simulink model "IOControls"  (R2019b)
settings: configuration reference "ConfigSet_IOControls_Reference" (kept outside this file)
model workspace (MAT data in the model file):
  SampleTime = 0.05
libraries: IOStateMachinesLib x274, SignalGeneratorsLib x1, simulink x1
(part 8 of 10)

== system IOControls/ForEachVehicle/IOControls/Non-CabControl/InteriorDoorControls/LeftDoor2ManualClose ==
  note: States:
      | Close
      | Open
  InputControl : Inport  OutDataTypeStr=Bus: BD_IOControls_In_InputControl
  Initialise : Inport  Port=2
  Bus Selector : BusSelector  OutputSignals=Value,Mode,InitVal,InternalRequest,Inhibit
  LeftDoor2ManualClose-Momentary : IOStateMachinesLib/Momentary  InitSource=internal  InitState=InitState
      settings: SourceProductName=IO State Machines
  InputState : Outport  VectorParamsAs1DForOutWhenUnconnected=off
  wires:
  Initialise/1 -> LeftDoor2ManualClose-Momentary/4
  LeftDoor2ManualClose-Momentary/1 -> InputState/1
  Bus Selector/5 -> LeftDoor2ManualClose-Momentary/6  "<Inhibit>"
  Bus Selector/4 -> LeftDoor2ManualClose-Momentary/5  "<InternalRequest>"
  Bus Selector/3 -> LeftDoor2ManualClose-Momentary/3  "<InitVal>"
  Bus Selector/2 -> LeftDoor2ManualClose-Momentary/2  "<Mode>"
  Bus Selector/1 -> LeftDoor2ManualClose-Momentary/1  "<Value>"
  InputControl/1 -> Bus Selector/1

== system IOControls/ForEachVehicle/IOControls/Non-CabControl/InteriorDoorControls/LeftDoor2ManualOpen ==
  note: States:
      | Close
      | Open
  InputControl : Inport  OutDataTypeStr=Bus: BD_IOControls_In_InputControl
  Initialise : Inport  Port=2
  Bus Selector : BusSelector  OutputSignals=Value,Mode,InitVal,InternalRequest,Inhibit
  LeftDoor2ManualOpen-Momentary : IOStateMachinesLib/Momentary  InitSource=internal  InitState=InitState
      settings: SourceProductName=IO State Machines
  InputState : Outport  VectorParamsAs1DForOutWhenUnconnected=off
  wires:
  Initialise/1 -> LeftDoor2ManualOpen-Momentary/4
  LeftDoor2ManualOpen-Momentary/1 -> InputState/1
  Bus Selector/5 -> LeftDoor2ManualOpen-Momentary/6  "<Inhibit>"
  Bus Selector/4 -> LeftDoor2ManualOpen-Momentary/5  "<InternalRequest>"
  Bus Selector/3 -> LeftDoor2ManualOpen-Momentary/3  "<InitVal>"
  Bus Selector/2 -> LeftDoor2ManualOpen-Momentary/2  "<Mode>"
  Bus Selector/1 -> LeftDoor2ManualOpen-Momentary/1  "<Value>"
  InputControl/1 -> Bus Selector/1

== system IOControls/ForEachVehicle/IOControls/Non-CabControl/InteriorDoorControls/LeftDoor3Coving ==
  note: States:
      | Closed
      | Open
  InputControl : Inport  OutDataTypeStr=Bus: BD_IOControls_In_InputControl
  Initialise : Inport  Port=2
  Bus Selector : BusSelector  OutputSignals=Value,Mode,InitVal,InternalRequest,Inhibit
  LeftDoor3Coving-Toggle : IOStateMachinesLib/Toggle  InitSource=internal  InitState=InitState  OffStateValue=OffStateValue  OnStateValue=OnStateValue
      settings: SourceProductName=IO State Machines
  InputState : Outport  VectorParamsAs1DForOutWhenUnconnected=off
  wires:
  Initialise/1 -> LeftDoor3Coving-Toggle/4
  LeftDoor3Coving-Toggle/1 -> InputState/1
  Bus Selector/5 -> LeftDoor3Coving-Toggle/6  "<Inhibit>"
  Bus Selector/4 -> LeftDoor3Coving-Toggle/5  "<InternalRequest>"
  Bus Selector/3 -> LeftDoor3Coving-Toggle/3  "<InitVal>"
  Bus Selector/2 -> LeftDoor3Coving-Toggle/2  "<Mode>"
  Bus Selector/1 -> LeftDoor3Coving-Toggle/1  "<Value>"
  InputControl/1 -> Bus Selector/1

== system IOControls/ForEachVehicle/IOControls/Non-CabControl/InteriorDoorControls/LeftDoor3DCUCB ==
  note: States:
      | Tripped
      | Set
  MCBControl : Inport  OutDataTypeStr=Bus: BD_IOControls_In_MCBControl
  Initialise : Inport  Port=2
  Bus Selector : BusSelector  OutputSignals=Value,Mode,InitVal,InternalRequest,Inhibit,TripRequest
  LeftDoor3DCUCB-MCB : IOStateMachinesLib/MCB  InitSource=internal  InitState=InitState  OffStateValue=OffStateValue  OnStateValue=OnStateValue
      settings: SourceProductName=IO State Machines
  InputState : Outport  VectorParamsAs1DForOutWhenUnconnected=off
  MCBTripState : Outport  Port=2  VectorParamsAs1DForOutWhenUnconnected=off
  wires:
  LeftDoor3DCUCB-MCB/2 -> MCBTripState/1
  Bus Selector/6 -> LeftDoor3DCUCB-MCB/7  "<TripRequest>"
  MCBControl/1 -> Bus Selector/1
  Bus Selector/1 -> LeftDoor3DCUCB-MCB/1  "<Value>"
  Bus Selector/2 -> LeftDoor3DCUCB-MCB/2  "<Mode>"
  Bus Selector/3 -> LeftDoor3DCUCB-MCB/3  "<InitVal>"
  Bus Selector/4 -> LeftDoor3DCUCB-MCB/5  "<InternalRequest>"
  Bus Selector/5 -> LeftDoor3DCUCB-MCB/6  "<Inhibit>"
  LeftDoor3DCUCB-MCB/1 -> InputState/1
  Initialise/1 -> LeftDoor3DCUCB-MCB/4

== system IOControls/ForEachVehicle/IOControls/Non-CabControl/InteriorDoorControls/LeftDoor3EED ==
  note: States:
      | Reset
      | Operated
  InputControl : Inport  OutDataTypeStr=Bus: BD_IOControls_In_InputControl
  Initialise : Inport  Port=2
  Bus Selector : BusSelector  OutputSignals=Value,Mode,InitVal,InternalRequest,Inhibit
  LeftDoor3EED-Momentary : IOStateMachinesLib/Momentary  InitSource=internal  InitState=InitState
      settings: SourceProductName=IO State Machines
  InputState : Outport  VectorParamsAs1DForOutWhenUnconnected=off
  wires:
  Initialise/1 -> LeftDoor3EED-Momentary/4
  LeftDoor3EED-Momentary/1 -> InputState/1
  Bus Selector/5 -> LeftDoor3EED-Momentary/6  "<Inhibit>"
  Bus Selector/4 -> LeftDoor3EED-Momentary/5  "<InternalRequest>"
  Bus Selector/3 -> LeftDoor3EED-Momentary/3  "<InitVal>"
  Bus Selector/2 -> LeftDoor3EED-Momentary/2  "<Mode>"
  Bus Selector/1 -> LeftDoor3EED-Momentary/1  "<Value>"
  InputControl/1 -> Bus Selector/1

== system IOControls/ForEachVehicle/IOControls/Non-CabControl/InteriorDoorControls/LeftDoor3Lockout ==
  note: States:
      | Unlocked
      | Locked
  InputControl : Inport  OutDataTypeStr=Bus: BD_IOControls_In_InputControl
  Initialise : Inport  Port=2
  Bus Selector : BusSelector  OutputSignals=Value,Mode,InitVal,InternalRequest,Inhibit
  LeftDoor3Lockout-Toggle : IOStateMachinesLib/Toggle  InitSource=internal  InitState=InitState  OffStateValue=OffStateValue  OnStateValue=OnStateValue
      settings: SourceProductName=IO State Machines
  InputState : Outport  VectorParamsAs1DForOutWhenUnconnected=off
  wires:
  Initialise/1 -> LeftDoor3Lockout-Toggle/4
  LeftDoor3Lockout-Toggle/1 -> InputState/1
  Bus Selector/5 -> LeftDoor3Lockout-Toggle/6  "<Inhibit>"
  Bus Selector/4 -> LeftDoor3Lockout-Toggle/5  "<InternalRequest>"
  Bus Selector/3 -> LeftDoor3Lockout-Toggle/3  "<InitVal>"
  Bus Selector/2 -> LeftDoor3Lockout-Toggle/2  "<Mode>"
  Bus Selector/1 -> LeftDoor3Lockout-Toggle/1  "<Value>"
  InputControl/1 -> Bus Selector/1

== system IOControls/ForEachVehicle/IOControls/Non-CabControl/InteriorDoorControls/LeftDoor3ManualClose ==
  note: States:
      | Close
      | Open
  InputControl : Inport  OutDataTypeStr=Bus: BD_IOControls_In_InputControl
  Initialise : Inport  Port=2
  Bus Selector : BusSelector  OutputSignals=Value,Mode,InitVal,InternalRequest,Inhibit
  LeftDoor3ManualClose-Momentary : IOStateMachinesLib/Momentary  InitSource=internal  InitState=InitState
      settings: SourceProductName=IO State Machines
  InputState : Outport  VectorParamsAs1DForOutWhenUnconnected=off
  wires:
  Initialise/1 -> LeftDoor3ManualClose-Momentary/4
  LeftDoor3ManualClose-Momentary/1 -> InputState/1
  Bus Selector/5 -> LeftDoor3ManualClose-Momentary/6  "<Inhibit>"
  Bus Selector/4 -> LeftDoor3ManualClose-Momentary/5  "<InternalRequest>"
  Bus Selector/3 -> LeftDoor3ManualClose-Momentary/3  "<InitVal>"
  Bus Selector/2 -> LeftDoor3ManualClose-Momentary/2  "<Mode>"
  Bus Selector/1 -> LeftDoor3ManualClose-Momentary/1  "<Value>"
  InputControl/1 -> Bus Selector/1

== system IOControls/ForEachVehicle/IOControls/Non-CabControl/InteriorDoorControls/LeftDoor3ManualOpen ==
  note: States:
      | Close
      | Open
  InputControl : Inport  OutDataTypeStr=Bus: BD_IOControls_In_InputControl
  Initialise : Inport  Port=2
  Bus Selector : BusSelector  OutputSignals=Value,Mode,InitVal,InternalRequest,Inhibit
  LeftDoor3ManualOpen-Momentary : IOStateMachinesLib/Momentary  InitSource=internal  InitState=InitState
      settings: SourceProductName=IO State Machines
  InputState : Outport  VectorParamsAs1DForOutWhenUnconnected=off
  wires:
  Initialise/1 -> LeftDoor3ManualOpen-Momentary/4
  LeftDoor3ManualOpen-Momentary/1 -> InputState/1
  Bus Selector/5 -> LeftDoor3ManualOpen-Momentary/6  "<Inhibit>"
  Bus Selector/4 -> LeftDoor3ManualOpen-Momentary/5  "<InternalRequest>"
  Bus Selector/3 -> LeftDoor3ManualOpen-Momentary/3  "<InitVal>"
  Bus Selector/2 -> LeftDoor3ManualOpen-Momentary/2  "<Mode>"
  Bus Selector/1 -> LeftDoor3ManualOpen-Momentary/1  "<Value>"
  InputControl/1 -> Bus Selector/1

== system IOControls/ForEachVehicle/IOControls/Non-CabControl/InteriorDoorControls/LeftDoor4Coving ==
  note: States:
      | Closed
      | Open
  InputControl : Inport  OutDataTypeStr=Bus: BD_IOControls_In_InputControl
  Initialise : Inport  Port=2
  Bus Selector : BusSelector  OutputSignals=Value,Mode,InitVal,InternalRequest,Inhibit
  LeftDoor4Coving-Toggle : IOStateMachinesLib/Toggle  InitSource=internal  InitState=InitState  OffStateValue=OffStateValue  OnStateValue=OnStateValue
      settings: SourceProductName=IO State Machines
  InputState : Outport  VectorParamsAs1DForOutWhenUnconnected=off
  wires:
  Initialise/1 -> LeftDoor4Coving-Toggle/4
  LeftDoor4Coving-Toggle/1 -> InputState/1
  Bus Selector/5 -> LeftDoor4Coving-Toggle/6  "<Inhibit>"
  Bus Selector/4 -> LeftDoor4Coving-Toggle/5  "<InternalRequest>"
  Bus Selector/3 -> LeftDoor4Coving-Toggle/3  "<InitVal>"
  Bus Selector/2 -> LeftDoor4Coving-Toggle/2  "<Mode>"
  Bus Selector/1 -> LeftDoor4Coving-Toggle/1  "<Value>"
  InputControl/1 -> Bus Selector/1

== system IOControls/ForEachVehicle/IOControls/Non-CabControl/InteriorDoorControls/LeftDoor4DCUCB ==
  note: States:
      | Tripped
      | Set
  MCBControl : Inport  OutDataTypeStr=Bus: BD_IOControls_In_MCBControl
  Initialise : Inport  Port=2
  Bus Selector : BusSelector  OutputSignals=Value,Mode,InitVal,InternalRequest,Inhibit,TripRequest
  LeftDoor4DCUCB-MCB : IOStateMachinesLib/MCB  InitSource=internal  InitState=InitState  OffStateValue=OffStateValue  OnStateValue=OnStateValue
      settings: SourceProductName=IO State Machines
  InputState : Outport  VectorParamsAs1DForOutWhenUnconnected=off
  MCBTripState : Outport  Port=2  VectorParamsAs1DForOutWhenUnconnected=off
  wires:
  LeftDoor4DCUCB-MCB/2 -> MCBTripState/1
  Bus Selector/6 -> LeftDoor4DCUCB-MCB/7  "<TripRequest>"
  MCBControl/1 -> Bus Selector/1
  Bus Selector/1 -> LeftDoor4DCUCB-MCB/1  "<Value>"
  Bus Selector/2 -> LeftDoor4DCUCB-MCB/2  "<Mode>"
  Bus Selector/3 -> LeftDoor4DCUCB-MCB/3  "<InitVal>"
  Bus Selector/4 -> LeftDoor4DCUCB-MCB/5  "<InternalRequest>"
  Bus Selector/5 -> LeftDoor4DCUCB-MCB/6  "<Inhibit>"
  LeftDoor4DCUCB-MCB/1 -> InputState/1
  Initialise/1 -> LeftDoor4DCUCB-MCB/4

== system IOControls/ForEachVehicle/IOControls/Non-CabControl/InteriorDoorControls/LeftDoor4EED ==
  note: States:
      | Reset
      | Operated
  InputControl : Inport  OutDataTypeStr=Bus: BD_IOControls_In_InputControl
  Initialise : Inport  Port=2
  Bus Selector : BusSelector  OutputSignals=Value,Mode,InitVal,InternalRequest,Inhibit
  LeftDoor4EED-Momentary : IOStateMachinesLib/Momentary  InitSource=internal  InitState=InitState
      settings: SourceProductName=IO State Machines
  InputState : Outport  VectorParamsAs1DForOutWhenUnconnected=off
  wires:
  Initialise/1 -> LeftDoor4EED-Momentary/4
  LeftDoor4EED-Momentary/1 -> InputState/1
  Bus Selector/5 -> LeftDoor4EED-Momentary/6  "<Inhibit>"
  Bus Selector/4 -> LeftDoor4EED-Momentary/5  "<InternalRequest>"
  Bus Selector/3 -> LeftDoor4EED-Momentary/3  "<InitVal>"
  Bus Selector/2 -> LeftDoor4EED-Momentary/2  "<Mode>"
  Bus Selector/1 -> LeftDoor4EED-Momentary/1  "<Value>"
  InputControl/1 -> Bus Selector/1

== system IOControls/ForEachVehicle/IOControls/Non-CabControl/InteriorDoorControls/LeftDoor4Lockout ==
  note: States:
      | Unlocked
      | Locked
  InputControl : Inport  OutDataTypeStr=Bus: BD_IOControls_In_InputControl
  Initialise : Inport  Port=2
  Bus Selector : BusSelector  OutputSignals=Value,Mode,InitVal,InternalRequest,Inhibit
  LeftDoor4Lockout-Toggle : IOStateMachinesLib/Toggle  InitSource=internal  InitState=InitState  OffStateValue=OffStateValue  OnStateValue=OnStateValue
      settings: SourceProductName=IO State Machines
  InputState : Outport  VectorParamsAs1DForOutWhenUnconnected=off
  wires:
  Initialise/1 -> LeftDoor4Lockout-Toggle/4
  LeftDoor4Lockout-Toggle/1 -> InputState/1
  Bus Selector/5 -> LeftDoor4Lockout-Toggle/6  "<Inhibit>"
  Bus Selector/4 -> LeftDoor4Lockout-Toggle/5  "<InternalRequest>"
  Bus Selector/3 -> LeftDoor4Lockout-Toggle/3  "<InitVal>"
  Bus Selector/2 -> LeftDoor4Lockout-Toggle/2  "<Mode>"
  Bus Selector/1 -> LeftDoor4Lockout-Toggle/1  "<Value>"
  InputControl/1 -> Bus Selector/1

== system IOControls/ForEachVehicle/IOControls/Non-CabControl/InteriorDoorControls/LeftDoor4ManualClose ==
  note: States:
      | Close
      | Open
  InputControl : Inport  OutDataTypeStr=Bus: BD_IOControls_In_InputControl
  Initialise : Inport  Port=2
  Bus Selector : BusSelector  OutputSignals=Value,Mode,InitVal,InternalRequest,Inhibit
  LeftDoor4ManualClose-Momentary : IOStateMachinesLib/Momentary  InitSource=internal  InitState=InitState
      settings: SourceProductName=IO State Machines
  InputState : Outport  VectorParamsAs1DForOutWhenUnconnected=off
  wires:
  Initialise/1 -> LeftDoor4ManualClose-Momentary/4
  LeftDoor4ManualClose-Momentary/1 -> InputState/1
  Bus Selector/5 -> LeftDoor4ManualClose-Momentary/6  "<Inhibit>"
  Bus Selector/4 -> LeftDoor4ManualClose-Momentary/5  "<InternalRequest>"
  Bus Selector/3 -> LeftDoor4ManualClose-Momentary/3  "<InitVal>"
  Bus Selector/2 -> LeftDoor4ManualClose-Momentary/2  "<Mode>"
  Bus Selector/1 -> LeftDoor4ManualClose-Momentary/1  "<Value>"
  InputControl/1 -> Bus Selector/1

== system IOControls/ForEachVehicle/IOControls/Non-CabControl/InteriorDoorControls/LeftDoor4ManualOpen ==
  note: States:
      | Close
      | Open
  InputControl : Inport  OutDataTypeStr=Bus: BD_IOControls_In_InputControl
  Initialise : Inport  Port=2
  Bus Selector : BusSelector  OutputSignals=Value,Mode,InitVal,InternalRequest,Inhibit
  LeftDoor4ManualOpen-Momentary : IOStateMachinesLib/Momentary  InitSource=internal  InitState=InitState
      settings: SourceProductName=IO State Machines
  InputState : Outport  VectorParamsAs1DForOutWhenUnconnected=off
  wires:
  Initialise/1 -> LeftDoor4ManualOpen-Momentary/4
  LeftDoor4ManualOpen-Momentary/1 -> InputState/1
  Bus Selector/5 -> LeftDoor4ManualOpen-Momentary/6  "<Inhibit>"
  Bus Selector/4 -> LeftDoor4ManualOpen-Momentary/5  "<InternalRequest>"
  Bus Selector/3 -> LeftDoor4ManualOpen-Momentary/3  "<InitVal>"
  Bus Selector/2 -> LeftDoor4ManualOpen-Momentary/2  "<Mode>"
  Bus Selector/1 -> LeftDoor4ManualOpen-Momentary/1  "<Value>"
  InputControl/1 -> Bus Selector/1

== system IOControls/ForEachVehicle/IOControls/Non-CabControl/InteriorDoorControls/RightDoor1Coving ==
  note: States:
      | Closed
      | Open
  InputControl : Inport  OutDataTypeStr=Bus: BD_IOControls_In_InputControl
  Initialise : Inport  Port=2
  Bus Selector : BusSelector  OutputSignals=Value,Mode,InitVal,InternalRequest,Inhibit
  RightDoor1Coving-Toggle : IOStateMachinesLib/Toggle  InitSource=internal  InitState=InitState  OffStateValue=OffStateValue  OnStateValue=OnStateValue
      settings: SourceProductName=IO State Machines
  InputState : Outport  VectorParamsAs1DForOutWhenUnconnected=off
  wires:
  Initialise/1 -> RightDoor1Coving-Toggle/4
  RightDoor1Coving-Toggle/1 -> InputState/1
  Bus Selector/5 -> RightDoor1Coving-Toggle/6  "<Inhibit>"
  Bus Selector/4 -> RightDoor1Coving-Toggle/5  "<InternalRequest>"
  Bus Selector/3 -> RightDoor1Coving-Toggle/3  "<InitVal>"
  Bus Selector/2 -> RightDoor1Coving-Toggle/2  "<Mode>"
  Bus Selector/1 -> RightDoor1Coving-Toggle/1  "<Value>"
  InputControl/1 -> Bus Selector/1

== system IOControls/ForEachVehicle/IOControls/Non-CabControl/InteriorDoorControls/RightDoor1DCUCB ==
  note: States:
      | Tripped
      | Set
  MCBControl : Inport  OutDataTypeStr=Bus: BD_IOControls_In_MCBControl
  Initialise : Inport  Port=2
  Bus Selector : BusSelector  OutputSignals=Value,Mode,InitVal,InternalRequest,Inhibit,TripRequest
  RightDoor1DCUCB-MCB : IOStateMachinesLib/MCB  InitSource=internal  InitState=InitState  OffStateValue=OffStateValue  OnStateValue=OnStateValue
      settings: SourceProductName=IO State Machines
  InputState : Outport  VectorParamsAs1DForOutWhenUnconnected=off
  MCBTripState : Outport  Port=2  VectorParamsAs1DForOutWhenUnconnected=off
  wires:
  RightDoor1DCUCB-MCB/2 -> MCBTripState/1
  Bus Selector/6 -> RightDoor1DCUCB-MCB/7  "<TripRequest>"
  MCBControl/1 -> Bus Selector/1
  Bus Selector/1 -> RightDoor1DCUCB-MCB/1  "<Value>"
  Bus Selector/2 -> RightDoor1DCUCB-MCB/2  "<Mode>"
  Bus Selector/3 -> RightDoor1DCUCB-MCB/3  "<InitVal>"
  Bus Selector/4 -> RightDoor1DCUCB-MCB/5  "<InternalRequest>"
  Bus Selector/5 -> RightDoor1DCUCB-MCB/6  "<Inhibit>"
  RightDoor1DCUCB-MCB/1 -> InputState/1
  Initialise/1 -> RightDoor1DCUCB-MCB/4

== system IOControls/ForEachVehicle/IOControls/Non-CabControl/InteriorDoorControls/RightDoor1EED ==
  note: States:
      | Reset
      | Operated
  InputControl : Inport  OutDataTypeStr=Bus: BD_IOControls_In_InputControl
  Initialise : Inport  Port=2
  Bus Selector : BusSelector  OutputSignals=Value,Mode,InitVal,InternalRequest,Inhibit
  RightDoor1EED-Momentary : IOStateMachinesLib/Momentary  InitSource=internal  InitState=InitState
      settings: SourceProductName=IO State Machines
  InputState : Outport  VectorParamsAs1DForOutWhenUnconnected=off
  wires:
  Initialise/1 -> RightDoor1EED-Momentary/4
  RightDoor1EED-Momentary/1 -> InputState/1
  Bus Selector/5 -> RightDoor1EED-Momentary/6  "<Inhibit>"
  Bus Selector/4 -> RightDoor1EED-Momentary/5  "<InternalRequest>"
  Bus Selector/3 -> RightDoor1EED-Momentary/3  "<InitVal>"
  Bus Selector/2 -> RightDoor1EED-Momentary/2  "<Mode>"
  Bus Selector/1 -> RightDoor1EED-Momentary/1  "<Value>"
  InputControl/1 -> Bus Selector/1

== system IOControls/ForEachVehicle/IOControls/Non-CabControl/InteriorDoorControls/RightDoor1Lockout ==
  note: States:
      | Unlocked
      | Locked
  InputControl : Inport  OutDataTypeStr=Bus: BD_IOControls_In_InputControl
  Initialise : Inport  Port=2
  Bus Selector : BusSelector  OutputSignals=Value,Mode,InitVal,InternalRequest,Inhibit
  RightDoor1Lockout-Toggle : IOStateMachinesLib/Toggle  InitSource=internal  InitState=InitState  OffStateValue=OffStateValue  OnStateValue=OnStateValue
      settings: SourceProductName=IO State Machines
  InputState : Outport  VectorParamsAs1DForOutWhenUnconnected=off
  wires:
  Initialise/1 -> RightDoor1Lockout-Toggle/4
  RightDoor1Lockout-Toggle/1 -> InputState/1
  Bus Selector/5 -> RightDoor1Lockout-Toggle/6  "<Inhibit>"
  Bus Selector/4 -> RightDoor1Lockout-Toggle/5  "<InternalRequest>"
  Bus Selector/3 -> RightDoor1Lockout-Toggle/3  "<InitVal>"
  Bus Selector/2 -> RightDoor1Lockout-Toggle/2  "<Mode>"
  Bus Selector/1 -> RightDoor1Lockout-Toggle/1  "<Value>"
  InputControl/1 -> Bus Selector/1

== system IOControls/ForEachVehicle/IOControls/Non-CabControl/InteriorDoorControls/RightDoor1ManualClose ==
  note: States:
      | Close
      | Open
  InputControl : Inport  OutDataTypeStr=Bus: BD_IOControls_In_InputControl
  Initialise : Inport  Port=2
  Bus Selector : BusSelector  OutputSignals=Value,Mode,InitVal,InternalRequest,Inhibit
  RightDoor1ManualClose-Momentary : IOStateMachinesLib/Momentary  InitSource=internal  InitState=InitState
      settings: SourceProductName=IO State Machines
  InputState : Outport  VectorParamsAs1DForOutWhenUnconnected=off
  wires:
  Initialise/1 -> RightDoor1ManualClose-Momentary/4
  RightDoor1ManualClose-Momentary/1 -> InputState/1
  Bus Selector/5 -> RightDoor1ManualClose-Momentary/6  "<Inhibit>"
  Bus Selector/4 -> RightDoor1ManualClose-Momentary/5  "<InternalRequest>"
  Bus Selector/3 -> RightDoor1ManualClose-Momentary/3  "<InitVal>"
  Bus Selector/2 -> RightDoor1ManualClose-Momentary/2  "<Mode>"
  Bus Selector/1 -> RightDoor1ManualClose-Momentary/1  "<Value>"
  InputControl/1 -> Bus Selector/1

== system IOControls/ForEachVehicle/IOControls/Non-CabControl/InteriorDoorControls/RightDoor1ManualOpen ==
  note: States:
      | Close
      | Open
  InputControl : Inport  OutDataTypeStr=Bus: BD_IOControls_In_InputControl
  Initialise : Inport  Port=2
  Bus Selector : BusSelector  OutputSignals=Value,Mode,InitVal,InternalRequest,Inhibit
  RightDoor1ManualOpen-Momentary : IOStateMachinesLib/Momentary  InitSource=internal  InitState=InitState
      settings: SourceProductName=IO State Machines
  InputState : Outport  VectorParamsAs1DForOutWhenUnconnected=off
  wires:
  Initialise/1 -> RightDoor1ManualOpen-Momentary/4
  RightDoor1ManualOpen-Momentary/1 -> InputState/1
  Bus Selector/5 -> RightDoor1ManualOpen-Momentary/6  "<Inhibit>"
  Bus Selector/4 -> RightDoor1ManualOpen-Momentary/5  "<InternalRequest>"
  Bus Selector/3 -> RightDoor1ManualOpen-Momentary/3  "<InitVal>"
  Bus Selector/2 -> RightDoor1ManualOpen-Momentary/2  "<Mode>"
  Bus Selector/1 -> RightDoor1ManualOpen-Momentary/1  "<Value>"
  InputControl/1 -> Bus Selector/1

== system IOControls/ForEachVehicle/IOControls/Non-CabControl/InteriorDoorControls/RightDoor2Coving ==
  note: States:
      | Closed
      | Open
  InputControl : Inport  OutDataTypeStr=Bus: BD_IOControls_In_InputControl
  Initialise : Inport  Port=2
  Bus Selector : BusSelector  OutputSignals=Value,Mode,InitVal,InternalRequest,Inhibit
  RightDoor2Coving-Toggle : IOStateMachinesLib/Toggle  InitSource=internal  InitState=InitState  OffStateValue=OffStateValue  OnStateValue=OnStateValue
      settings: SourceProductName=IO State Machines
  InputState : Outport  VectorParamsAs1DForOutWhenUnconnected=off
  wires:
  Initialise/1 -> RightDoor2Coving-Toggle/4
  RightDoor2Coving-Toggle/1 -> InputState/1
  Bus Selector/5 -> RightDoor2Coving-Toggle/6  "<Inhibit>"
  Bus Selector/4 -> RightDoor2Coving-Toggle/5  "<InternalRequest>"
  Bus Selector/3 -> RightDoor2Coving-Toggle/3  "<InitVal>"
  Bus Selector/2 -> RightDoor2Coving-Toggle/2  "<Mode>"
  Bus Selector/1 -> RightDoor2Coving-Toggle/1  "<Value>"
  InputControl/1 -> Bus Selector/1

== system IOControls/ForEachVehicle/IOControls/Non-CabControl/InteriorDoorControls/RightDoor2DCUCB ==
  note: States:
      | Tripped
      | Set
  MCBControl : Inport  OutDataTypeStr=Bus: BD_IOControls_In_MCBControl
  Initialise : Inport  Port=2
  Bus Selector : BusSelector  OutputSignals=Value,Mode,InitVal,InternalRequest,Inhibit,TripRequest
  RightDoor2DCUCB-MCB : IOStateMachinesLib/MCB  InitSource=internal  InitState=InitState  OffStateValue=OffStateValue  OnStateValue=OnStateValue
      settings: SourceProductName=IO State Machines
  InputState : Outport  VectorParamsAs1DForOutWhenUnconnected=off
  MCBTripState : Outport  Port=2  VectorParamsAs1DForOutWhenUnconnected=off
  wires:
  RightDoor2DCUCB-MCB/2 -> MCBTripState/1
  Bus Selector/6 -> RightDoor2DCUCB-MCB/7  "<TripRequest>"
  MCBControl/1 -> Bus Selector/1
  Bus Selector/1 -> RightDoor2DCUCB-MCB/1  "<Value>"
  Bus Selector/2 -> RightDoor2DCUCB-MCB/2  "<Mode>"
  Bus Selector/3 -> RightDoor2DCUCB-MCB/3  "<InitVal>"
  Bus Selector/4 -> RightDoor2DCUCB-MCB/5  "<InternalRequest>"
  Bus Selector/5 -> RightDoor2DCUCB-MCB/6  "<Inhibit>"
  RightDoor2DCUCB-MCB/1 -> InputState/1
  Initialise/1 -> RightDoor2DCUCB-MCB/4

== system IOControls/ForEachVehicle/IOControls/Non-CabControl/InteriorDoorControls/RightDoor2EED ==
  note: States:
      | Reset
      | Operated
  InputControl : Inport  OutDataTypeStr=Bus: BD_IOControls_In_InputControl
  Initialise : Inport  Port=2
  Bus Selector : BusSelector  OutputSignals=Value,Mode,InitVal,InternalRequest,Inhibit
  RightDoor2EED-Momentary : IOStateMachinesLib/Momentary  InitSource=internal  InitState=InitState
      settings: SourceProductName=IO State Machines
  InputState : Outport  VectorParamsAs1DForOutWhenUnconnected=off
  wires:
  Initialise/1 -> RightDoor2EED-Momentary/4
  RightDoor2EED-Momentary/1 -> InputState/1
  Bus Selector/5 -> RightDoor2EED-Momentary/6  "<Inhibit>"
  Bus Selector/4 -> RightDoor2EED-Momentary/5  "<InternalRequest>"
  Bus Selector/3 -> RightDoor2EED-Momentary/3  "<InitVal>"
  Bus Selector/2 -> RightDoor2EED-Momentary/2  "<Mode>"
  Bus Selector/1 -> RightDoor2EED-Momentary/1  "<Value>"
  InputControl/1 -> Bus Selector/1

== system IOControls/ForEachVehicle/IOControls/Non-CabControl/InteriorDoorControls/RightDoor2Lockout ==
  note: States:
      | Unlocked
      | Locked
  InputControl : Inport  OutDataTypeStr=Bus: BD_IOControls_In_InputControl
  Initialise : Inport  Port=2
  Bus Selector : BusSelector  OutputSignals=Value,Mode,InitVal,InternalRequest,Inhibit
  RightDoor2Lockout-Toggle : IOStateMachinesLib/Toggle  InitSource=internal  InitState=InitState  OffStateValue=OffStateValue  OnStateValue=OnStateValue
      settings: SourceProductName=IO State Machines
  InputState : Outport  VectorParamsAs1DForOutWhenUnconnected=off
  wires:
  Initialise/1 -> RightDoor2Lockout-Toggle/4
  RightDoor2Lockout-Toggle/1 -> InputState/1
  Bus Selector/5 -> RightDoor2Lockout-Toggle/6  "<Inhibit>"
  Bus Selector/4 -> RightDoor2Lockout-Toggle/5  "<InternalRequest>"
  Bus Selector/3 -> RightDoor2Lockout-Toggle/3  "<InitVal>"
  Bus Selector/2 -> RightDoor2Lockout-Toggle/2  "<Mode>"
  Bus Selector/1 -> RightDoor2Lockout-Toggle/1  "<Value>"
  InputControl/1 -> Bus Selector/1

== system IOControls/ForEachVehicle/IOControls/Non-CabControl/InteriorDoorControls/RightDoor2ManualClose ==
  note: States:
      | Close
      | Open
  InputControl : Inport  OutDataTypeStr=Bus: BD_IOControls_In_InputControl
  Initialise : Inport  Port=2
  Bus Selector : BusSelector  OutputSignals=Value,Mode,InitVal,InternalRequest,Inhibit
  RightDoor2ManualClose-Momentary : IOStateMachinesLib/Momentary  InitSource=internal  InitState=InitState
      settings: SourceProductName=IO State Machines
  InputState : Outport  VectorParamsAs1DForOutWhenUnconnected=off
  wires:
  Initialise/1 -> RightDoor2ManualClose-Momentary/4
  RightDoor2ManualClose-Momentary/1 -> InputState/1
  Bus Selector/5 -> RightDoor2ManualClose-Momentary/6  "<Inhibit>"
  Bus Selector/4 -> RightDoor2ManualClose-Momentary/5  "<InternalRequest>"
  Bus Selector/3 -> RightDoor2ManualClose-Momentary/3  "<InitVal>"
  Bus Selector/2 -> RightDoor2ManualClose-Momentary/2  "<Mode>"
  Bus Selector/1 -> RightDoor2ManualClose-Momentary/1  "<Value>"
  InputControl/1 -> Bus Selector/1

== system IOControls/ForEachVehicle/IOControls/Non-CabControl/InteriorDoorControls/RightDoor2ManualOpen ==
  note: States:
      | Close
      | Open
  InputControl : Inport  OutDataTypeStr=Bus: BD_IOControls_In_InputControl
  Initialise : Inport  Port=2
  Bus Selector : BusSelector  OutputSignals=Value,Mode,InitVal,InternalRequest,Inhibit
  RightDoor2ManualOpen-Momentary : IOStateMachinesLib/Momentary  InitSource=internal  InitState=InitState
      settings: SourceProductName=IO State Machines
  InputState : Outport  VectorParamsAs1DForOutWhenUnconnected=off
  wires:
  Initialise/1 -> RightDoor2ManualOpen-Momentary/4
  RightDoor2ManualOpen-Momentary/1 -> InputState/1
  Bus Selector/5 -> RightDoor2ManualOpen-Momentary/6  "<Inhibit>"
  Bus Selector/4 -> RightDoor2ManualOpen-Momentary/5  "<InternalRequest>"
  Bus Selector/3 -> RightDoor2ManualOpen-Momentary/3  "<InitVal>"
  Bus Selector/2 -> RightDoor2ManualOpen-Momentary/2  "<Mode>"
  Bus Selector/1 -> RightDoor2ManualOpen-Momentary/1  "<Value>"
  InputControl/1 -> Bus Selector/1

== system IOControls/ForEachVehicle/IOControls/Non-CabControl/InteriorDoorControls/RightDoor3Coving ==
  note: States:
      | Closed
      | Open
  InputControl : Inport  OutDataTypeStr=Bus: BD_IOControls_In_InputControl
  Initialise : Inport  Port=2
  Bus Selector : BusSelector  OutputSignals=Value,Mode,InitVal,InternalRequest,Inhibit
  RightDoor3Coving-Toggle : IOStateMachinesLib/Toggle  InitSource=internal  InitState=InitState  OffStateValue=OffStateValue  OnStateValue=OnStateValue
      settings: SourceProductName=IO State Machines
  InputState : Outport  VectorParamsAs1DForOutWhenUnconnected=off
  wires:
  Initialise/1 -> RightDoor3Coving-Toggle/4
  RightDoor3Coving-Toggle/1 -> InputState/1
  Bus Selector/5 -> RightDoor3Coving-Toggle/6  "<Inhibit>"
  Bus Selector/4 -> RightDoor3Coving-Toggle/5  "<InternalRequest>"
  Bus Selector/3 -> RightDoor3Coving-Toggle/3  "<InitVal>"
  Bus Selector/2 -> RightDoor3Coving-Toggle/2  "<Mode>"
  Bus Selector/1 -> RightDoor3Coving-Toggle/1  "<Value>"
  InputControl/1 -> Bus Selector/1

== system IOControls/ForEachVehicle/IOControls/Non-CabControl/InteriorDoorControls/RightDoor3DCUCB ==
  note: States:
      | Tripped
      | Set
  MCBControl : Inport  OutDataTypeStr=Bus: BD_IOControls_In_MCBControl
  Initialise : Inport  Port=2
  Bus Selector : BusSelector  OutputSignals=Value,Mode,InitVal,InternalRequest,Inhibit,TripRequest
  RightDoor3DCUCB-MCB : IOStateMachinesLib/MCB  InitSource=internal  InitState=InitState  OffStateValue=OffStateValue  OnStateValue=OnStateValue
      settings: SourceProductName=IO State Machines
  InputState : Outport  VectorParamsAs1DForOutWhenUnconnected=off
  MCBTripState : Outport  Port=2  VectorParamsAs1DForOutWhenUnconnected=off
  wires:
  RightDoor3DCUCB-MCB/2 -> MCBTripState/1
  Bus Selector/6 -> RightDoor3DCUCB-MCB/7  "<TripRequest>"
  MCBControl/1 -> Bus Selector/1
  Bus Selector/1 -> RightDoor3DCUCB-MCB/1  "<Value>"
  Bus Selector/2 -> RightDoor3DCUCB-MCB/2  "<Mode>"
  Bus Selector/3 -> RightDoor3DCUCB-MCB/3  "<InitVal>"
  Bus Selector/4 -> RightDoor3DCUCB-MCB/5  "<InternalRequest>"
  Bus Selector/5 -> RightDoor3DCUCB-MCB/6  "<Inhibit>"
  RightDoor3DCUCB-MCB/1 -> InputState/1
  Initialise/1 -> RightDoor3DCUCB-MCB/4

== system IOControls/ForEachVehicle/IOControls/Non-CabControl/InteriorDoorControls/RightDoor3EED ==
  note: States:
      | Reset
      | Operated
  InputControl : Inport  OutDataTypeStr=Bus: BD_IOControls_In_InputControl
  Initialise : Inport  Port=2
  Bus Selector : BusSelector  OutputSignals=Value,Mode,InitVal,InternalRequest,Inhibit
  RightDoor3EED-Momentary : IOStateMachinesLib/Momentary  InitSource=internal  InitState=InitState
      settings: SourceProductName=IO State Machines
  InputState : Outport  VectorParamsAs1DForOutWhenUnconnected=off
  wires:
  Initialise/1 -> RightDoor3EED-Momentary/4
  RightDoor3EED-Momentary/1 -> InputState/1
  Bus Selector/5 -> RightDoor3EED-Momentary/6  "<Inhibit>"
  Bus Selector/4 -> RightDoor3EED-Momentary/5  "<InternalRequest>"
  Bus Selector/3 -> RightDoor3EED-Momentary/3  "<InitVal>"
  Bus Selector/2 -> RightDoor3EED-Momentary/2  "<Mode>"
  Bus Selector/1 -> RightDoor3EED-Momentary/1  "<Value>"
  InputControl/1 -> Bus Selector/1

== system IOControls/ForEachVehicle/IOControls/Non-CabControl/InteriorDoorControls/RightDoor3Lockout ==
  note: States:
      | Unlocked
      | Locked
  InputControl : Inport  OutDataTypeStr=Bus: BD_IOControls_In_InputControl
  Initialise : Inport  Port=2
  Bus Selector : BusSelector  OutputSignals=Value,Mode,InitVal,InternalRequest,Inhibit
  RightDoor3Lockout-Toggle : IOStateMachinesLib/Toggle  InitSource=internal  InitState=InitState  OffStateValue=OffStateValue  OnStateValue=OnStateValue
      settings: SourceProductName=IO State Machines
  InputState : Outport  VectorParamsAs1DForOutWhenUnconnected=off
  wires:
  Initialise/1 -> RightDoor3Lockout-Toggle/4
  RightDoor3Lockout-Toggle/1 -> InputState/1
  Bus Selector/5 -> RightDoor3Lockout-Toggle/6  "<Inhibit>"
  Bus Selector/4 -> RightDoor3Lockout-Toggle/5  "<InternalRequest>"
  Bus Selector/3 -> RightDoor3Lockout-Toggle/3  "<InitVal>"
  Bus Selector/2 -> RightDoor3Lockout-Toggle/2  "<Mode>"
  Bus Selector/1 -> RightDoor3Lockout-Toggle/1  "<Value>"
  InputControl/1 -> Bus Selector/1

== system IOControls/ForEachVehicle/IOControls/Non-CabControl/InteriorDoorControls/RightDoor3ManualClose ==
  note: States:
      | Close
      | Open
  InputControl : Inport  OutDataTypeStr=Bus: BD_IOControls_In_InputControl
  Initialise : Inport  Port=2
  Bus Selector : BusSelector  OutputSignals=Value,Mode,InitVal,InternalRequest,Inhibit
  RightDoor3ManualClose-Momentary : IOStateMachinesLib/Momentary  InitSource=internal  InitState=InitState
      settings: SourceProductName=IO State Machines
  InputState : Outport  VectorParamsAs1DForOutWhenUnconnected=off
  wires:
  Initialise/1 -> RightDoor3ManualClose-Momentary/4
  RightDoor3ManualClose-Momentary/1 -> InputState/1
  Bus Selector/5 -> RightDoor3ManualClose-Momentary/6  "<Inhibit>"
  Bus Selector/4 -> RightDoor3ManualClose-Momentary/5  "<InternalRequest>"
  Bus Selector/3 -> RightDoor3ManualClose-Momentary/3  "<InitVal>"
  Bus Selector/2 -> RightDoor3ManualClose-Momentary/2  "<Mode>"
  Bus Selector/1 -> RightDoor3ManualClose-Momentary/1  "<Value>"
  InputControl/1 -> Bus Selector/1

== system IOControls/ForEachVehicle/IOControls/Non-CabControl/InteriorDoorControls/RightDoor3ManualOpen ==
  note: States:
      | Close
      | Open
  InputControl : Inport  OutDataTypeStr=Bus: BD_IOControls_In_InputControl
  Initialise : Inport  Port=2
  Bus Selector : BusSelector  OutputSignals=Value,Mode,InitVal,InternalRequest,Inhibit
  RightDoor3ManualOpen-Momentary : IOStateMachinesLib/Momentary  InitSource=internal  InitState=InitState
      settings: SourceProductName=IO State Machines
  InputState : Outport  VectorParamsAs1DForOutWhenUnconnected=off
  wires:
  Initialise/1 -> RightDoor3ManualOpen-Momentary/4
  RightDoor3ManualOpen-Momentary/1 -> InputState/1
  Bus Selector/5 -> RightDoor3ManualOpen-Momentary/6  "<Inhibit>"
  Bus Selector/4 -> RightDoor3ManualOpen-Momentary/5  "<InternalRequest>"
  Bus Selector/3 -> RightDoor3ManualOpen-Momentary/3  "<InitVal>"
  Bus Selector/2 -> RightDoor3ManualOpen-Momentary/2  "<Mode>"
  Bus Selector/1 -> RightDoor3ManualOpen-Momentary/1  "<Value>"
  InputControl/1 -> Bus Selector/1

== system IOControls/ForEachVehicle/IOControls/Non-CabControl/InteriorDoorControls/RightDoor4Coving ==
  note: States:
      | Closed
      | Open
  InputControl : Inport  OutDataTypeStr=Bus: BD_IOControls_In_InputControl
  Initialise : Inport  Port=2
  Bus Selector : BusSelector  OutputSignals=Value,Mode,InitVal,InternalRequest,Inhibit
  RightDoor4Coving-Toggle : IOStateMachinesLib/Toggle  InitSource=internal  InitState=InitState  OffStateValue=OffStateValue  OnStateValue=OnStateValue
      settings: SourceProductName=IO State Machines
  InputState : Outport  VectorParamsAs1DForOutWhenUnconnected=off
  wires:
  Initialise/1 -> RightDoor4Coving-Toggle/4
  RightDoor4Coving-Toggle/1 -> InputState/1
  Bus Selector/5 -> RightDoor4Coving-Toggle/6  "<Inhibit>"
  Bus Selector/4 -> RightDoor4Coving-Toggle/5  "<InternalRequest>"
  Bus Selector/3 -> RightDoor4Coving-Toggle/3  "<InitVal>"
  Bus Selector/2 -> RightDoor4Coving-Toggle/2  "<Mode>"
  Bus Selector/1 -> RightDoor4Coving-Toggle/1  "<Value>"
  InputControl/1 -> Bus Selector/1

== system IOControls/ForEachVehicle/IOControls/Non-CabControl/InteriorDoorControls/RightDoor4DCUCB ==
  note: States:
      | Tripped
      | Set
  MCBControl : Inport  OutDataTypeStr=Bus: BD_IOControls_In_MCBControl
  Initialise : Inport  Port=2
  Bus Selector : BusSelector  OutputSignals=Value,Mode,InitVal,InternalRequest,Inhibit,TripRequest
  RightDoor4DCUCB-MCB : IOStateMachinesLib/MCB  InitSource=internal  InitState=InitState  OffStateValue=OffStateValue  OnStateValue=OnStateValue
      settings: SourceProductName=IO State Machines
  InputState : Outport  VectorParamsAs1DForOutWhenUnconnected=off
  MCBTripState : Outport  Port=2  VectorParamsAs1DForOutWhenUnconnected=off
  wires:
  RightDoor4DCUCB-MCB/2 -> MCBTripState/1
  Bus Selector/6 -> RightDoor4DCUCB-MCB/7  "<TripRequest>"
  MCBControl/1 -> Bus Selector/1
  Bus Selector/1 -> RightDoor4DCUCB-MCB/1  "<Value>"
  Bus Selector/2 -> RightDoor4DCUCB-MCB/2  "<Mode>"
  Bus Selector/3 -> RightDoor4DCUCB-MCB/3  "<InitVal>"
  Bus Selector/4 -> RightDoor4DCUCB-MCB/5  "<InternalRequest>"
  Bus Selector/5 -> RightDoor4DCUCB-MCB/6  "<Inhibit>"
  RightDoor4DCUCB-MCB/1 -> InputState/1
  Initialise/1 -> RightDoor4DCUCB-MCB/4

== system IOControls/ForEachVehicle/IOControls/Non-CabControl/InteriorDoorControls/RightDoor4EED ==
  note: States:
      | Reset
      | Operated
  InputControl : Inport  OutDataTypeStr=Bus: BD_IOControls_In_InputControl
  Initialise : Inport  Port=2
  Bus Selector : BusSelector  OutputSignals=Value,Mode,InitVal,InternalRequest,Inhibit
  RightDoor4EED-Momentary : IOStateMachinesLib/Momentary  InitSource=internal  InitState=InitState
      settings: SourceProductName=IO State Machines
  InputState : Outport  VectorParamsAs1DForOutWhenUnconnected=off
  wires:
  Initialise/1 -> RightDoor4EED-Momentary/4
  RightDoor4EED-Momentary/1 -> InputState/1
  Bus Selector/5 -> RightDoor4EED-Momentary/6  "<Inhibit>"
  Bus Selector/4 -> RightDoor4EED-Momentary/5  "<InternalRequest>"
  Bus Selector/3 -> RightDoor4EED-Momentary/3  "<InitVal>"
  Bus Selector/2 -> RightDoor4EED-Momentary/2  "<Mode>"
  Bus Selector/1 -> RightDoor4EED-Momentary/1  "<Value>"
  InputControl/1 -> Bus Selector/1

== system IOControls/ForEachVehicle/IOControls/Non-CabControl/InteriorDoorControls/RightDoor4Lockout ==
  note: States:
      | Unlocked
      | Locked
  InputControl : Inport  OutDataTypeStr=Bus: BD_IOControls_In_InputControl
  Initialise : Inport  Port=2
  Bus Selector : BusSelector  OutputSignals=Value,Mode,InitVal,InternalRequest,Inhibit
  RightDoor4Lockout-Toggle : IOStateMachinesLib/Toggle  InitSource=internal  InitState=InitState  OffStateValue=OffStateValue  OnStateValue=OnStateValue
      settings: SourceProductName=IO State Machines
  InputState : Outport  VectorParamsAs1DForOutWhenUnconnected=off
  wires:
  Initialise/1 -> RightDoor4Lockout-Toggle/4
  RightDoor4Lockout-Toggle/1 -> InputState/1
  Bus Selector/5 -> RightDoor4Lockout-Toggle/6  "<Inhibit>"
  Bus Selector/4 -> RightDoor4Lockout-Toggle/5  "<InternalRequest>"
  Bus Selector/3 -> RightDoor4Lockout-Toggle/3  "<InitVal>"
  Bus Selector/2 -> RightDoor4Lockout-Toggle/2  "<Mode>"
  Bus Selector/1 -> RightDoor4Lockout-Toggle/1  "<Value>"
  InputControl/1 -> Bus Selector/1

== system IOControls/ForEachVehicle/IOControls/Non-CabControl/InteriorDoorControls/RightDoor4ManualClose ==
  note: States:
      | Close
      | Open
  InputControl : Inport  OutDataTypeStr=Bus: BD_IOControls_In_InputControl
  Initialise : Inport  Port=2
  Bus Selector : BusSelector  OutputSignals=Value,Mode,InitVal,InternalRequest,Inhibit
  RightDoor4ManualClose-Momentary : IOStateMachinesLib/Momentary  InitSource=internal  InitState=InitState
      settings: SourceProductName=IO State Machines
  InputState : Outport  VectorParamsAs1DForOutWhenUnconnected=off
  wires:
  Initialise/1 -> RightDoor4ManualClose-Momentary/4
  RightDoor4ManualClose-Momentary/1 -> InputState/1
  Bus Selector/5 -> RightDoor4ManualClose-Momentary/6  "<Inhibit>"
  Bus Selector/4 -> RightDoor4ManualClose-Momentary/5  "<InternalRequest>"
  Bus Selector/3 -> RightDoor4ManualClose-Momentary/3  "<InitVal>"
  Bus Selector/2 -> RightDoor4ManualClose-Momentary/2  "<Mode>"
  Bus Selector/1 -> RightDoor4ManualClose-Momentary/1  "<Value>"
  InputControl/1 -> Bus Selector/1

== system IOControls/ForEachVehicle/IOControls/Non-CabControl/InteriorDoorControls/RightDoor4ManualOpen ==
  note: States:
      | Close
      | Open
  InputControl : Inport  OutDataTypeStr=Bus: BD_IOControls_In_InputControl
  Initialise : Inport  Port=2
  Bus Selector : BusSelector  OutputSignals=Value,Mode,InitVal,InternalRequest,Inhibit
  RightDoor4ManualOpen-Momentary : IOStateMachinesLib/Momentary  InitSource=internal  InitState=InitState
      settings: SourceProductName=IO State Machines
  InputState : Outport  VectorParamsAs1DForOutWhenUnconnected=off
  wires:
  Initialise/1 -> RightDoor4ManualOpen-Momentary/4
  RightDoor4ManualOpen-Momentary/1 -> InputState/1
  Bus Selector/5 -> RightDoor4ManualOpen-Momentary/6  "<Inhibit>"
  Bus Selector/4 -> RightDoor4ManualOpen-Momentary/5  "<InternalRequest>"
  Bus Selector/3 -> RightDoor4ManualOpen-Momentary/3  "<InitVal>"
  Bus Selector/2 -> RightDoor4ManualOpen-Momentary/2  "<Mode>"
  Bus Selector/1 -> RightDoor4ManualOpen-Momentary/1  "<Value>"
  InputControl/1 -> Bus Selector/1

== system IOControls/ForEachVehicle/IOControls/Non-CabControl/PassengerEmergencyControlUnit/DriversBackDoor ==
  note: States:
      | Off
      | On
  InputControl : Inport  OutDataTypeStr=Bus: BD_IOControls_In_InputControl
  Initialise : Inport  Port=2
  Bus Selector : BusSelector  OutputSignals=Value,Mode,InitVal,InternalRequest,Inhibit
  DriversBackDoor-Toggle : IOStateMachinesLib/Toggle  InitSource=internal  InitState=InitState  OffStateValue=OffStateValue  OnStateValue=OnStateValue
      settings: SourceProductName=IO State Machines
  InputState : Outport  VectorParamsAs1DForOutWhenUnconnected=off
  wires:
  Initialise/1 -> DriversBackDoor-Toggle/4
  DriversBackDoor-Toggle/1 -> InputState/1
  Bus Selector/5 -> DriversBackDoor-Toggle/6  "<Inhibit>"
  Bus Selector/4 -> DriversBackDoor-Toggle/5  "<InternalRequest>"
  Bus Selector/3 -> DriversBackDoor-Toggle/3  "<InitVal>"
  Bus Selector/2 -> DriversBackDoor-Toggle/2  "<Mode>"
  Bus Selector/1 -> DriversBackDoor-Toggle/1  "<Value>"
  InputControl/1 -> Bus Selector/1

== system IOControls/ForEachVehicle/IOControls/Non-CabControl/PassengerEmergencyControlUnit/Microphone ==
  note: States:
      | Release
      | Push
  InputControl : Inport  OutDataTypeStr=Bus: BD_IOControls_In_InputControl
  Initialise : Inport  Port=2
  Bus Selector : BusSelector  OutputSignals=Value,Mode,InitVal,InternalRequest,Inhibit
  Microphone-Momentary : IOStateMachinesLib/Momentary  InitSource=internal  InitState=InitState
      settings: SourceProductName=IO State Machines
  InputState : Outport  VectorParamsAs1DForOutWhenUnconnected=off
  wires:
  Initialise/1 -> Microphone-Momentary/4
  Microphone-Momentary/1 -> InputState/1
  Bus Selector/5 -> Microphone-Momentary/6  "<Inhibit>"
  Bus Selector/4 -> Microphone-Momentary/5  "<InternalRequest>"
  Bus Selector/3 -> Microphone-Momentary/3  "<InitVal>"
  Bus Selector/2 -> Microphone-Momentary/2  "<Mode>"
  Bus Selector/1 -> Microphone-Momentary/1  "<Value>"
  InputControl/1 -> Bus Selector/1

== system IOControls/ForEachVehicle/IOControls/Non-CabControl/PassengerEmergencyControlUnit/PECUPushButton ==
  note: States:
      | Release
      | Push
  InputControl : Inport  OutDataTypeStr=Bus: BD_IOControls_In_InputControl
  Initialise : Inport  Port=2
  Bus Selector : BusSelector  OutputSignals=Value,Mode,InitVal,InternalRequest,Inhibit
  PECUPushButton-Momentary : IOStateMachinesLib/Momentary  InitSource=internal  InitState=InitState
      settings: SourceProductName=IO State Machines
  InputState : Outport  VectorParamsAs1DForOutWhenUnconnected=off
  wires:
  Initialise/1 -> PECUPushButton-Momentary/4
  PECUPushButton-Momentary/1 -> InputState/1
  Bus Selector/5 -> PECUPushButton-Momentary/6  "<Inhibit>"
  Bus Selector/4 -> PECUPushButton-Momentary/5  "<InternalRequest>"
  Bus Selector/3 -> PECUPushButton-Momentary/3  "<InitVal>"
  Bus Selector/2 -> PECUPushButton-Momentary/2  "<Mode>"
  Bus Selector/1 -> PECUPushButton-Momentary/1  "<Value>"
  InputControl/1 -> Bus Selector/1

== system IOControls/ForEachVehicle/IOControls/Non-CabControl/PneumaticControls/ASCOEnd1 ==
  note: States:
      | Isolated
      | Normal
  InputControl : Inport  OutDataTypeStr=Bus: BD_IOControls_In_InputControl
  Initialise : Inport  Port=2
  ASCOEnd1-Toggle : IOStateMachinesLib/Toggle  InitSource=internal  InitState=InitState  OffStateValue=OffStateValue  OnStateValue=OnStateValue
      settings: SourceProductName=IO State Machines
  Bus Selector : BusSelector  OutputSignals=Value,Mode,InitVal,InternalRequest,Inhibit
  InputState : Outport  VectorParamsAs1DForOutWhenUnconnected=off
  wires:
  Initialise/1 -> ASCOEnd1-Toggle/4
  ASCOEnd1-Toggle/1 -> InputState/1
  Bus Selector/5 -> ASCOEnd1-Toggle/6  "<Inhibit>"
  Bus Selector/4 -> ASCOEnd1-Toggle/5  "<InternalRequest>"
  Bus Selector/3 -> ASCOEnd1-Toggle/3  "<InitVal>"
  Bus Selector/2 -> ASCOEnd1-Toggle/2  "<Mode>"
  Bus Selector/1 -> ASCOEnd1-Toggle/1  "<Value>"
  InputControl/1 -> Bus Selector/1

== system IOControls/ForEachVehicle/IOControls/Non-CabControl/PneumaticControls/ASCOEnd2 ==
  note: States:
      | Isolated
      | Normal
  InputControl : Inport  OutDataTypeStr=Bus: BD_IOControls_In_InputControl
  Initialise : Inport  Port=2
  ASCOEnd2-Toggle : IOStateMachinesLib/Toggle  InitSource=internal  InitState=InitState  OffStateValue=OffStateValue  OnStateValue=OnStateValue
      settings: SourceProductName=IO State Machines
  Bus Selector : BusSelector  OutputSignals=Value,Mode,InitVal,InternalRequest,Inhibit
  InputState : Outport  VectorParamsAs1DForOutWhenUnconnected=off
  wires:
  Initialise/1 -> ASCOEnd2-Toggle/4
  ASCOEnd2-Toggle/1 -> InputState/1
  Bus Selector/5 -> ASCOEnd2-Toggle/6  "<Inhibit>"
  Bus Selector/4 -> ASCOEnd2-Toggle/5  "<InternalRequest>"
  Bus Selector/3 -> ASCOEnd2-Toggle/3  "<InitVal>"
  Bus Selector/2 -> ASCOEnd2-Toggle/2  "<Mode>"
  Bus Selector/1 -> ASCOEnd2-Toggle/1  "<Value>"
  InputControl/1 -> Bus Selector/1

== system IOControls/ForEachVehicle/IOControls/Non-CabControl/PneumaticControls/ASIsolationCock ==
  note: States:
      | Isolated
      | Normal
  InputControl : Inport  OutDataTypeStr=Bus: BD_IOControls_In_InputControl
  Initialise : Inport  Port=2
  ASIsolationCock-Toggle : IOStateMachinesLib/Toggle  InitSource=internal  InitState=InitState  OffStateValue=OffStateValue  OnStateValue=OnStateValue
      settings: SourceProductName=IO State Machines
  Bus Selector : BusSelector  OutputSignals=Value,Mode,InitVal,InternalRequest,Inhibit
  InputState : Outport  VectorParamsAs1DForOutWhenUnconnected=off
  wires:
  Initialise/1 -> ASIsolationCock-Toggle/4
  ASIsolationCock-Toggle/1 -> InputState/1
  Bus Selector/5 -> ASIsolationCock-Toggle/6  "<Inhibit>"
  Bus Selector/4 -> ASIsolationCock-Toggle/5  "<InternalRequest>"
  Bus Selector/3 -> ASIsolationCock-Toggle/3  "<InitVal>"
  Bus Selector/2 -> ASIsolationCock-Toggle/2  "<Mode>"
  Bus Selector/1 -> ASIsolationCock-Toggle/1  "<Value>"
  InputControl/1 -> Bus Selector/1

== system IOControls/ForEachVehicle/IOControls/Non-CabControl/PneumaticControls/BIC1Inside ==
  note: States:
      | Isolated
      | Normal
  InputControl : Inport  OutDataTypeStr=Bus: BD_IOControls_In_InputControl
  Initialise : Inport  Port=2
  BIC1Inside-Toggle : IOStateMachinesLib/Toggle  InitSource=internal  InitState=InitState  OffStateValue=OffStateValue  OnStateValue=OnStateValue
      settings: SourceProductName=IO State Machines
  Bus Selector : BusSelector  OutputSignals=Value,Mode,InitVal,InternalRequest,Inhibit
  InputState : Outport  VectorParamsAs1DForOutWhenUnconnected=off
  wires:
  Initialise/1 -> BIC1Inside-Toggle/4
  BIC1Inside-Toggle/1 -> InputState/1
  Bus Selector/5 -> BIC1Inside-Toggle/6  "<Inhibit>"
  Bus Selector/4 -> BIC1Inside-Toggle/5  "<InternalRequest>"
  Bus Selector/3 -> BIC1Inside-Toggle/3  "<InitVal>"
  Bus Selector/2 -> BIC1Inside-Toggle/2  "<Mode>"
  Bus Selector/1 -> BIC1Inside-Toggle/1  "<Value>"
  InputControl/1 -> Bus Selector/1

== system IOControls/ForEachVehicle/IOControls/Non-CabControl/PneumaticControls/BIC1Outside ==
  note: States:
      | Isolated
      | Normal
  InputControl : Inport  OutDataTypeStr=Bus: BD_IOControls_In_InputControl
  Initialise : Inport  Port=2
  BIC1Outside-Toggle : IOStateMachinesLib/Toggle  InitSource=internal  InitState=InitState  OffStateValue=OffStateValue  OnStateValue=OnStateValue
      settings: SourceProductName=IO State Machines
  Bus Selector : BusSelector  OutputSignals=Value,Mode,InitVal,InternalRequest,Inhibit
  InputState : Outport  VectorParamsAs1DForOutWhenUnconnected=off
  wires:
  Initialise/1 -> BIC1Outside-Toggle/4
  BIC1Outside-Toggle/1 -> InputState/1
  Bus Selector/5 -> BIC1Outside-Toggle/6  "<Inhibit>"
  Bus Selector/4 -> BIC1Outside-Toggle/5  "<InternalRequest>"
  Bus Selector/3 -> BIC1Outside-Toggle/3  "<InitVal>"
  Bus Selector/2 -> BIC1Outside-Toggle/2  "<Mode>"
  Bus Selector/1 -> BIC1Outside-Toggle/1  "<Value>"
  InputControl/1 -> Bus Selector/1

== system IOControls/ForEachVehicle/IOControls/Non-CabControl/PneumaticControls/BIC2Inside ==
  note: States:
      | Isolated
      | Normal
  InputControl : Inport  OutDataTypeStr=Bus: BD_IOControls_In_InputControl
  Initialise : Inport  Port=2
  BIC2Inside-Toggle : IOStateMachinesLib/Toggle  InitSource=internal  InitState=InitState  OffStateValue=OffStateValue  OnStateValue=OnStateValue
      settings: SourceProductName=IO State Machines
  Bus Selector : BusSelector  OutputSignals=Value,Mode,InitVal,InternalRequest,Inhibit
  InputState : Outport  VectorParamsAs1DForOutWhenUnconnected=off
  wires:
  Initialise/1 -> BIC2Inside-Toggle/4
  BIC2Inside-Toggle/1 -> InputState/1
  Bus Selector/5 -> BIC2Inside-Toggle/6  "<Inhibit>"
  Bus Selector/4 -> BIC2Inside-Toggle/5  "<InternalRequest>"
  Bus Selector/3 -> BIC2Inside-Toggle/3  "<InitVal>"
  Bus Selector/2 -> BIC2Inside-Toggle/2  "<Mode>"
  Bus Selector/1 -> BIC2Inside-Toggle/1  "<Value>"
  InputControl/1 -> Bus Selector/1

== system IOControls/ForEachVehicle/IOControls/Non-CabControl/PneumaticControls/BIC2Outside ==
  note: States:
      | Isolated
      | Normal
  InputControl : Inport  OutDataTypeStr=Bus: BD_IOControls_In_InputControl
  Initialise : Inport  Port=2
  BIC2Outside-Toggle : IOStateMachinesLib/Toggle  InitSource=internal  InitState=InitState  OffStateValue=OffStateValue  OnStateValue=OnStateValue
      settings: SourceProductName=IO State Machines
  Bus Selector : BusSelector  OutputSignals=Value,Mode,InitVal,InternalRequest,Inhibit
  InputState : Outport  VectorParamsAs1DForOutWhenUnconnected=off
  wires:
  Initialise/1 -> BIC2Outside-Toggle/4
  BIC2Outside-Toggle/1 -> InputState/1
  Bus Selector/5 -> BIC2Outside-Toggle/6  "<Inhibit>"
  Bus Selector/4 -> BIC2Outside-Toggle/5  "<InternalRequest>"
  Bus Selector/3 -> BIC2Outside-Toggle/3  "<InitVal>"
  Bus Selector/2 -> BIC2Outside-Toggle/2  "<Mode>"
  Bus Selector/1 -> BIC2Outside-Toggle/1  "<Value>"
  InputControl/1 -> Bus Selector/1
